simulink model "XY_2mm_accelcontrol"  (R2023a)
settings: Solver=ode1  StartTime=0.0  StopTime=inf  FixedStep=0.001  RelTol=1e-3  EnableMultiTasking=on
PostLoadFcn:
  | , if any(exist('dsrtsu_mdlpostloadfcn', 'file') ~= 0), dsrtsu_mdlpostloadfcn('Execute', bdroot); end,
InitFcn:
  | , if any(exist('rtifpga_mdlclblib', 'file') ~= 0), rtifpga_mdlclblib('Init', bdroot); end,
  | [b,a] = butter(6,0.6)
  | N_coils = 6
  | % Load mean voltage needed for stationary levitation at "center" for the ML model's given dataset
  | load("D:\Maglev_Project\00_WORKSTATION\MATLAB Training\alldata.mat","Vmean_raw")
  | tic
model workspace (MAT data in the model file):
  Iters = 5
  N_coils = 6
  fatness_default = 1
  running = 0
  z0_default = 0.080001
undefined symbols (not defined in the file or in its folder): a, b, DiscIntNeverNeededParam, Vmean_raw
libraries: neural x15, simulink x8, commfilt2 x7, dspstat3 x4, rti2004lib x3, rtilibm x1
(part 1 of 3)
settings Model: DSRTSU_INTERNAL_RTI_VER=620  DSRTSU_INTERNAL_RTI_TYPE=rti1006  DSRTSU_INTERNAL_RTIFPGA=200  DSRTSU_INTERNAL_RTISTBM_VER=23.1  Creator=Administrator  LastModifiedBy=inst
settings SolverCC: AlgebraicLoopSolver=TrustRegion
settings DataIOCC: LimitDataPoints=on  SaveFormat=Array  SignalLoggingSaveFormat=ModelDataLogs  ReturnWorkspaceOutputs=off
settings OptimizationCC: BlockReduction=off  OptimizeBlockIOStorage=off  BufferReuse=off  ReuseModelBlockBuffer=off  ExpressionFolding=off  ExpressionDepthLimit=2147483647  LocalBlockOutputs=off  LifeSpan=inf
settings DebuggingCC: UnderspecifiedInitializationDetection=Classic  MergeDetectMultiDrivingBlocksExec=none  SolverPrmCheckMsg=warning  FcnCallInpInsideContextMsg=warning  UnconnectedInputMsg=warning  UnconnectedOutputMsg=warning  UnconnectedLineMsg=warning  StateNameClashWarn=warning  SFUnexpectedBacktrackingDiag=warning  SFNoUnconditionalDefaultTransitionDiag=warning  SFExecutionAtInitializationDiag=none  ArithmeticOperatorsInVariantConditions=warning
settings HardwareCC: ProdBitPerPointer=32  ProdBitPerSizeT=32  ProdBitPerPtrDiffT=32  ProdLargestAtomicInteger=Integer  ProdWordSize=32  ProdHWDeviceType=Custom Processor->Custom  TargetIntDivRoundTo=Zero  TargetEndianess=LittleEndian  TargetHWDeviceType=Custom Processor->Custom
settings ModelReferenceCC: EnableRefExpFcnMdlSchedulingChecks=on  PropagateSignalLabelsOutOfModel=off
settings SFSimCC: SimUseLocalCustomCode=off  MATLABDynamicMemAlloc=off  CustomCodeUndefinedFunction=UseInterfaceOnly
settings RTWCC: Description=dSPACE DS1006 Hardware Platform  SystemTargetFile=rti1006.tlc  MakeCommand=make_rti  TemplateMakefile=rti1006.tmf  RTWUseLocalCustomCode=off
settings CodeAppCC: StateflowObjectComments=on
settings STFCustomTargetCC: TargetLangStandard=C89/C90 (ANSI)  ParMdlRefBuildCompliant=on  ConcurrentExecutionCompliant=off  GRTInterface=off  UseToolchainInfoCompliant=off  SystemTargetFile=rti1006.tlc
settings GRTTargetCC: TargetLangStandard=C89/C90 (ANSI)  CompOptLevelCompliant=off  ConcurrentExecutionCompliant=off  CombineOutputUpdateFcns=off  MatFileLogging=off  CPPClassGenCompliant=off  UseToolchainInfoCompliant=off  ExtModeMexFile=noextcomm
settings ConfigComp: CovMetricSettings=dw  CovSaveCumulativeToWorkspaceVar=on  CovSaveSingleToWorkspaceVar=on

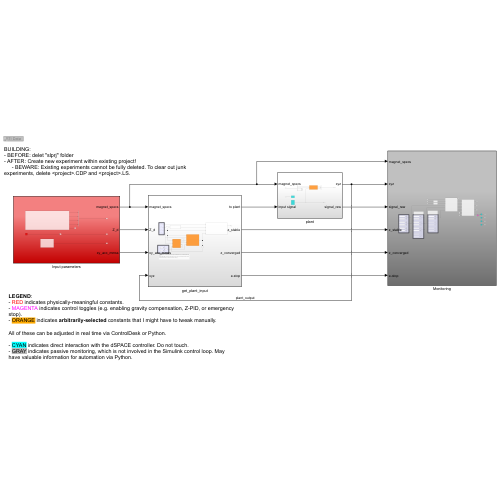
[thumbnail: Simulink's stored preview of the top-level diagram]
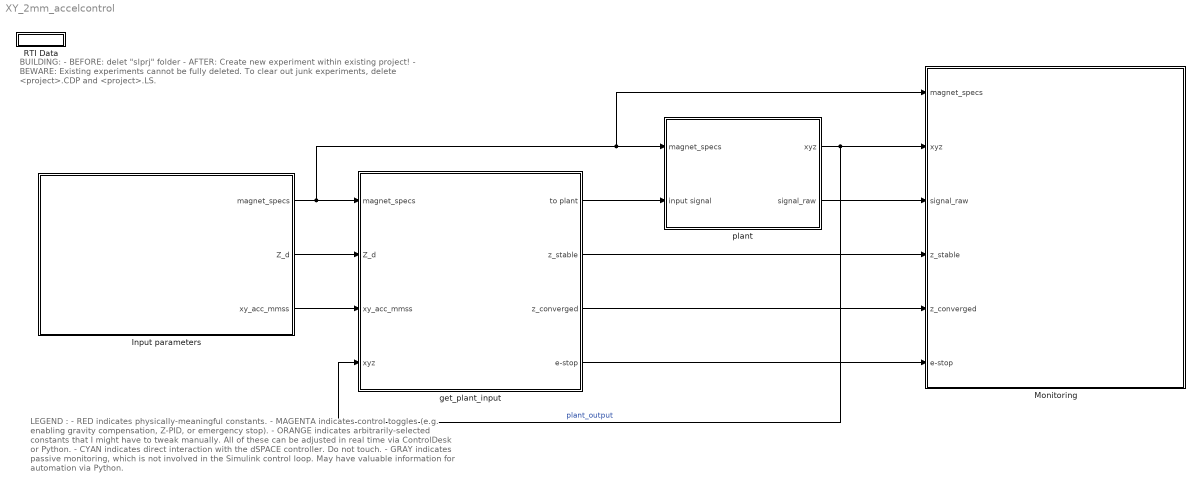
== system XY_2mm_accelcontrol ==
  note: BUILDING:
      | - BEFORE: delet "slprj" folder
      | - AFTER: Create new experiment within existing project!
      | - BEWARE: Existing experiments cannot be fully deleted. To clear out junk experiments, delete <project>.CDP and <project>.LS.
  note: LEGEND :
      | - RED indicates physically-meaningful constants.
      | - MAGENTA indicates control toggles (e.g. enabling gravity compensation, Z-PID, or emergency stop).
      | - ORANGE indicates arbitrarily-selected constants that I might have to tweak manually.
      |
      | All of these can be adjusted in real time via ControlDesk or Python.
      |
      | - CYAN indicates direct interaction with the dSPACE controller. Do not touch.
      | - GRAY indicates passive monitoring, which is not involved in the Simulink control loop. May have valuable information for automation via Python.
  Input parameters : Subsystem
  Monitoring : Subsystem
  RTI Data : Subsystem  Tag=struct('RTIDataServer',struct('RTIDataServerVs','2','RTIModelDescription','struct(''main'',''XY_2mm_accelcontrol'',''sub'','''',''isMp'',0)'))  LoadFcn="if exist('rtidc'), try,  rtidc('DataHostBlockClbLoad', gcbh); catch, disp(['Warning: ''LoadFcn'' for RTI Data block failed: ' lasterr]); end, end,"  mask(RTI_DATA_HOST){}
      mask help:
      | RTI Data Block.
      | This block is used by RTI to store internal model-dependent data.
      | Please keep this block on the root level of the model. Deleting this block will result in data loss.
      |
      | NEVER DELETE OR COPY THIS BLOCK!
      settings: CopyFcn="if exist('rtidc'), try,  rtidc('DataHostBlockClbCopy', gcbh); catch, disp(['Warning: ''CopyFcn'' for RTI Data block failed: ' lasterr]); end, end,"  DeleteFcn="if exist('rtidc'), try,  rtidc('DataHostBlockClbDelete', gcbh); catch, disp(['Warning: ''DeleteFcn'' for RTI Data block failed: ' lasterr]); end, end,"  ModelCloseFcn="if exist('rtidc'), try,  rtidc('DataHostBlockClbModelClose', gcbh); catch, disp(['Warning: ''ModelCloseFcn'' for RTI Data block failed: ' lasterr]); end, end,"  PreSaveFcn="if exist('rtidc'), try,  rtidc('DataHostBlockClbPreSave', gcbh); catch, disp(['Warning: ''PreSaveFcn'' for RTI Data block failed: ' lasterr]); end, end,"  PostSaveFcn="if exist('rtidc'), try,  rtidc('DataHostBlockClbPostSave', gcbh); catch, disp(['Warning: ''PostSaveFcn'' for RTI Data block failed: ' lasterr]); end, end,"  NameChangeFcn="if exist('rtidc'), try,  rtidc('DataHostBlockClbNameChange', gcbh); catch, disp(['Warning: ''NameChangeFcn'' for RTI Data block failed: ' lasterr]); end, end,"
      mask Help:
      | RTI Data Block.
      | This block is used by RTI to store internal model-dependent data.
      | Please keep this block on the root level of the model. Deleting this block will result in data loss.
      | 
      | NEVER DELETE OR COPY THIS BLOCK!
      mask Display:
      | text(0.5, 0.5, 'RTI Data', 'HorizontalAlignment', 'center');
      | plot([1 0]);
  get_plant_input : Subsystem
  plant : Subsystem
  wires:
  Input parameters/1(magnet_specs) -> Monitoring/1(magnet_specs), plant/1(magnet_specs), get_plant_input/1(magnet_specs)
  Input parameters/2(Z_d) -> get_plant_input/2(Z_d)
  plant/1(xyz) -> get_plant_input/4(xyz), Monitoring/2(xyz)  "plant_output"
  Input parameters/3(xy_acc_mmss) -> get_plant_input/3(xy_acc_mmss)
  get_plant_input/1(to plant) -> plant/2(input signal)
  plant/2(signal_raw) -> Monitoring/3(signal_raw)
  get_plant_input/2(z_stable) -> Monitoring/4(z_stable)
  get_plant_input/3(z_converged) -> Monitoring/5(z_converged)
  get_plant_input/4(e-stop) -> Monitoring/6(e-stop)

== system XY_2mm_accelcontrol/Input parameters ==
  Acceleration input : Subsystem
  Magnet Specs : Subsystem
  Mux : Mux
  Terminator : Terminator
  Z_desired_true : Constant  Value=0
  gain_dummy : Gain
  magnet_specs : Outport
  Z_d : Outport  Port=2
  xy_acc_mmss : Outport  Port=3
  wires:
  Magnet Specs/1(diameter_m) -> Mux/1
  Magnet Specs/2(height_m) -> Mux/2
  Magnet Specs/3(mass_g) -> Mux/3
  Magnet Specs/4(B_r) -> Mux/4
  Mux/1 -> magnet_specs/1
  Magnet Specs/5(errorflag) -> Terminator/1
  Z_desired_true/1 -> gain_dummy/1  "Z_d_true_test_inputparameters"
  gain_dummy/1 -> Z_d/1  "Z_d_test_dummygain"
  Acceleration input/1(xy_acc_mmss) -> xy_acc_mmss/1

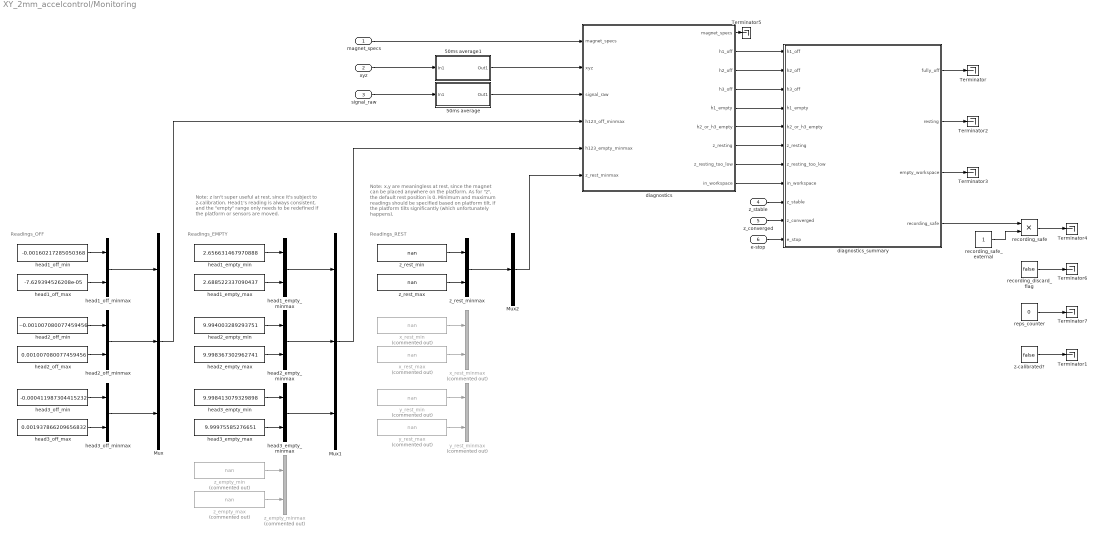
== system XY_2mm_accelcontrol/Monitoring ==
  note: Note: x,y are meaningless at rest, since the magnet can be placed anywhere on the platform.
      |
      | As for "z", the default rest position is 0. Minimum and maximum readings should be specified based on platform tilt, if the platform tilts significantly (which unfortunately happens).
  note: Readings_OFF
  note: Readings_REST
  note: Readings_EMPTY
  note: Note: z isn't super useful at rest, since it's subject to z-calibration.
      | Head1's reading is always consistent, and the "empty" range only needs to be redefined if the platform or sensors are moved.
  magnet_specs : Inport
  xyz : Inport  Port=2
  signal_raw : Inport  Port=3
  z_stable : Inport  Port=4
  z_converged : Inport  Port=5
  e-stop : Inport  Port=6
  50ms average : Subsystem
  50ms average1 : Subsystem
  Mux : Mux  Inputs=3
  Mux1 : Mux  Inputs=3
  Mux2 : Mux  Inputs=1
  Terminator{,1..7} (8 alike) : Terminator
  diagnostics : MATLAB Function  TreatAsAtomicUnit=on
  diagnostics_summary : MATLAB Function  TreatAsAtomicUnit=on
  head1_empty_max : Constant  Value=2.688522337090437
  head1_empty_min : Constant  Value=2.656631467970888
  head1_empty_minmax : Mux  Inputs=2
  head1_off_max : Constant  Value=-7.629394526208e-05
  head1_off_min : Constant  Value=-0.00160217285050368
  head1_off_minmax : Mux  Inputs=2
  head2_empty_max : Constant  Value=9.998367302962741
  head2_empty_min : Constant  Value=9.994003289293751
  head2_empty_minmax : Mux  Inputs=2
  head2_off_max : Constant  Value=0.001007080077459456
  head2_off_min : Constant  Value=--0.001007080077459456
  head2_off_minmax : Mux  Inputs=2
  head3_empty_max : Constant  Value=9.99975585276651
  head3_empty_min : Constant  Value=9.998413079329898
  head3_empty_minmax : Mux  Inputs=2
  head3_off_max : Constant  Value=0.001937866209656832
  head3_off_min : Constant  Value=-0.000411987304415232
  head3_off_minmax : Mux  Inputs=2
  recording_discard_flag : Constant  Value=false
  recording_safe : Product
  recording_safe_external : Constant
  reps_counter : Constant  Value=0
  x_rest_max : Constant  Commented=on  Value=nan
  x_rest_min : Constant  Commented=on  Value=nan
  x_rest_minmax : Mux  Commented=on  Inputs=2
  y_rest_max : Constant  Commented=on  Value=nan
  y_rest_min : Constant  Commented=on  Value=nan
  y_rest_minmax : Mux  Commented=on  Inputs=2
  z-calibrated? : Constant  Value=false
  z_empty_max : Constant  Commented=on  Value=nan
  z_empty_min : Constant  Commented=on  Value=nan
  z_empty_minmax : Mux  Commented=on  Inputs=2
  z_rest_max : Constant  Value=nan
  z_rest_min : Constant  Value=nan
  z_rest_minmax : Mux  Inputs=2
  wires:
  head1_off_min/1 -> head1_off_minmax/1
  head1_off_max/1 -> head1_off_minmax/2
  head2_off_min/1 -> head2_off_minmax/1
  head2_off_max/1 -> head2_off_minmax/2
  head3_off_max/1 -> head3_off_minmax/2
  head3_off_min/1 -> head3_off_minmax/1
  x_rest_max/1 -> x_rest_minmax/2
  z_rest_min/1 -> z_rest_minmax/1
  z_rest_max/1 -> z_rest_minmax/2
  y_rest_max/1 -> y_rest_minmax/2
  x_rest_min/1 -> x_rest_minmax/1
  y_rest_min/1 -> y_rest_minmax/1
  head3_empty_min/1 -> head3_empty_minmax/1
  head2_empty_min/1 -> head2_empty_minmax/1
  head3_empty_max/1 -> head3_empty_minmax/2
  head1_empty_min/1 -> head1_empty_minmax/1
  head2_empty_max/1 -> head2_empty_minmax/2
  head1_empty_max/1 -> head1_empty_minmax/2
  head1_off_minmax/1 -> Mux/1
  head2_off_minmax/1 -> Mux/2
  head3_off_minmax/1 -> Mux/3
  head2_empty_minmax/1 -> Mux1/2
  head3_empty_minmax/1 -> Mux1/3
  head1_empty_minmax/1 -> Mux1/1
  z_rest_minmax/1 -> Mux2/1
  Mux/1 -> diagnostics/4(h123_off_minmax)
  Mux1/1 -> diagnostics/5(h123_empty_minmax)
  Mux2/1 -> diagnostics/6(z_rest_minmax)
  z_empty_max/1 -> z_empty_minmax/2
  z_empty_min/1 -> z_empty_minmax/1
  magnet_specs/1 -> diagnostics/1("magnet_specs ")
  xyz/1 -> 50ms average1/1(In1)
  signal_raw/1 -> 50ms average/1(In1)
  z-calibrated?/1 -> Terminator1/1
  50ms average/1(Out1) -> diagnostics/3(signal_raw)
  50ms average1/1(Out1) -> diagnostics/2(xyz)
  diagnostics/2(h1_off) -> diagnostics_summary/1(h1_off)
  diagnostics/3(h2_off) -> diagnostics_summary/2(h2_off)
  diagnostics/4(h3_off) -> diagnostics_summary/3(h3_off)
  diagnostics/5(h1_empty) -> diagnostics_summary/4(h1_empty)
  diagnostics/6(h2_or_h3_empty) -> diagnostics_summary/5(h2_or_h3_empty)
  diagnostics/1(magnet_specs) -> Terminator5/1
  diagnostics/7(z_resting) -> diagnostics_summary/6(z_resting)
  diagnostics/8(z_resting_too_low) -> diagnostics_summary/7(z_resting_too_low)
  diagnostics/9(in_workspace) -> diagnostics_summary/8(in_workspace)
  diagnostics_summary/1(fully_off) -> Terminator/1
  diagnostics_summary/2(resting) -> Terminator2/1
  diagnostics_summary/3(empty_workspace) -> Terminator3/1
  diagnostics_summary/4(recording_safe) -> recording_safe/1
  z_converged/1 -> diagnostics_summary/10(z_converged)
  e-stop/1 -> diagnostics_summary/11(e_stop)
  recording_safe_external/1 -> recording_safe/2
  recording_safe/1 -> Terminator4/1
  z_stable/1 -> diagnostics_summary/9(z_stable)
  recording_discard_flag/1 -> Terminator6/1
  reps_counter/1 -> Terminator7/1

== system XY_2mm_accelcontrol/RTI Data ==
  RTI Data Store : Subsystem  Tag="struct('private',struct('version',struct('dsVer',uint32(2),'dsVerCreation',uint32(2),'RTI',struct('ver','6.2','type','RTI1006')),'access',struct('type','Model','isPerm',1,'created',['29-Jul-2010 10:53:51'],'modified',['20-Nov-2024 19:17:44'],'location','')),'public',struct('main',struct('data',[]),'sub',struct('name',{{'XY_2mm_accelcontrol'}},'data',{{struct('TH',struct('thTaskInfo',struct('taskType',{'TIMER','HWINT','TMRINT','SWINT','GLINT'},'tasksNumOf',{1,0,0,0,0},'srcIds',{{'TIMERA'},{},{},{},{}},'taskNames',{{['Timer Task 1']},{},{},{},{}})),'th_tc',struct('dataType','TASK','taskGroupId','','taskGroupList',{{}},'taskSchedulingPolicy','FCFS','taskType','TIMER','blkh',-1,'srcId','TIMERA','srcSgnName',['Timer A interrupt'],'srcCpuName','','taskName',['Timer Task 1  [0.001] s'],'taskNameDisplayExt','','smplTime',0.001,'smplTimeOffs',0,'hasFixedPriority',0,'priority',1,'hasFixedOvc',0,'ovcType',1,'ovcMax',1),'tc_th',struct('dataType','TASK','taskGroupId','','taskGroupList',{{}},'taskSchedulingPolicy','FCFS','taskType','TIMER','blkh',-1,'srcId','TIMERA','srcSgnName',['Timer A interrupt'],'srcCpuName','','taskName',['Timer Task 1  [0.001] s'],'taskNameDisplayExt','','smplTime',0.001,'smplTimeOffs',0,'hasFixedPriority',0,'priority',1,'hasFixedOvc',0,'ovcType',1,'ovcMax',1))}})))"  mask(RTI_DATA_STORE){}
      mask help:
      | RTI Data Store Block. This block is used by RTI to store internal model dependent data. Deleting this block will result in data loss.
      |
      | NEVER DELETE, COPY, OR MODIFY THIS BLOCK!
      mask Help:
      | RTI Data Store Block. This block is used by RTI to store internal model dependent data. Deleting this block will result in data loss.
      | 
      | NEVER DELETE, COPY, OR MODIFY THIS BLOCK!
      mask Display: text(0.5, 0.5, ' ', 'HorizontalAlignment', 'center');

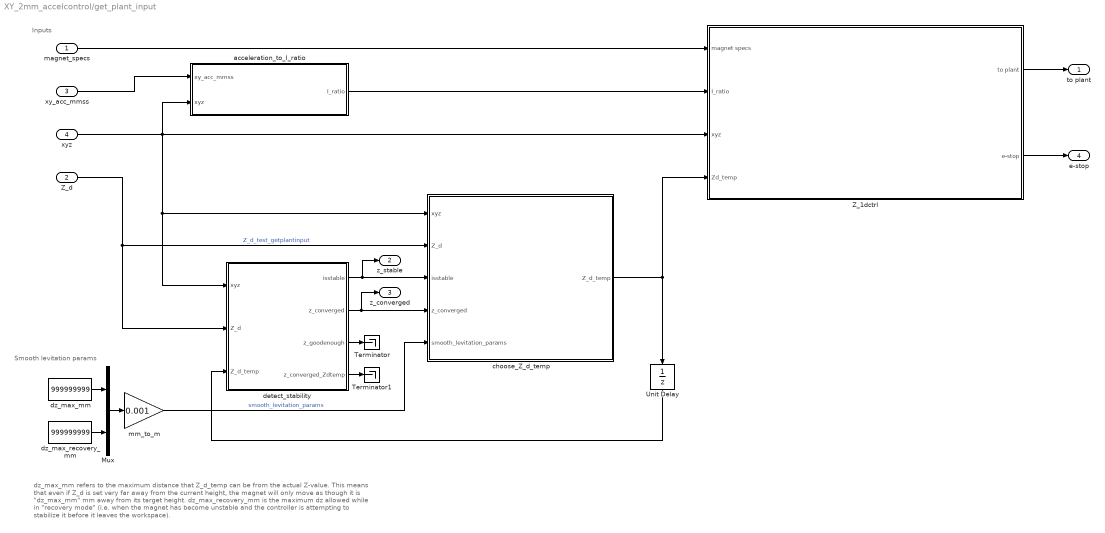
== system XY_2mm_accelcontrol/get_plant_input ==
  note: dz_max_mm refers to the maximum distance that Z_d_temp can be from the actual Z-value. This means that even if Z_d is set very far away from the current height, the magnet will only move as though it is "dz_max_mm" mm away from its target height.
      |
      | dz_max_recovery_mm is the maximum dz allowed while in "recovery mode" (i.e. when the magnet has become unstable and the controller is attempting to stabilize it before it leaves the workspace).
  note: Smooth levitation params
  note: Inputs
  magnet_specs : Inport
  Z_d : Inport  Port=2
  xy_acc_mmss : Inport  Port=3
  xyz : Inport  Port=4
  Mux : Mux  Inputs=2
  Terminator : Terminator
  Terminator1 : Terminator
  Unit Delay : UnitDelay  SampleTime=-1  HasFrameUpgradeWarning=on
  Z_1dctrl : Subsystem
  acceleration_to_I_ratio : Subsystem
  choose_Z_d_temp : Subsystem
  detect_stability : Subsystem
  dz_max_mm : Constant  Value=999999999
  dz_max_recovery_mm : Constant  Value=999999999
  mm_to_m : Gain  Gain=0.001
  to plant : Outport
  z_stable : Outport  Port=2
  z_converged : Outport  Port=3
  e-stop : Outport  Port=4
  wires:
  Z_d/1 -> detect_stability/2(Z_d), choose_Z_d_temp/2(Z_d)  "Z_d_test_getplantinput"
  xyz/1 -> acceleration_to_I_ratio/2(xyz), Z_1dctrl/3(xyz), detect_stability/1(xyz), choose_Z_d_temp/1(xyz)
  detect_stability/1(isstable) -> z_stable/1, choose_Z_d_temp/3(isstable)
  dz_max_mm/1 -> Mux/1
  dz_max_recovery_mm/1 -> Mux/2
  Mux/1 -> mm_to_m/1
  choose_Z_d_temp/1(Z_d_temp) -> Z_1dctrl/4(Zd_temp), Unit Delay/1
  detect_stability/2(z_converged) -> z_converged/1, choose_Z_d_temp/4(z_converged)
  detect_stability/3(z_goodenough) -> Terminator/1
  Unit Delay/1 -> detect_stability/3(Z_d_temp)
  Z_1dctrl/1(to plant) -> to plant/1
  magnet_specs/1 -> Z_1dctrl/1(magnet specs)
  xy_acc_mmss/1 -> acceleration_to_I_ratio/1(xy_acc_mmss)
  mm_to_m/1 -> choose_Z_d_temp/5(smooth_levitation_params)  "smooth_levitation_params"
  detect_stability/4(z_converged_Zdtemp) -> Terminator1/1
  Z_1dctrl/2(e-stop) -> e-stop/1
  acceleration_to_I_ratio/1(I_ratio) -> Z_1dctrl/2(I_ratio)

== system XY_2mm_accelcontrol/plant ==
  magnet_specs : Inport  PortDimensions=[1 4]
  input signal : Inport  Port=2
  DS2103_B1 : rtilibm/DS2103/DS2103_B1  BoardNo=1  ChannelNos=[1 2 4 6 8 9 10 11 12 18 19 20]  Range=[10 10 10 10 10 10 10 10 10 10 10 10 10 10 10 10 10 10 10 10 10 10 10 10 10 10 10 10 10 10 10 10]  IOErrorMode=[1 1 1 1 1 1 1 1]  InitValue=[0 0 0 0 0 0 0 0 0 0 0 0 0 0 0 0 0 0 0 0 0 0 0 0 0 0 0 0 0 0 0 0]  TermMode=[0 0 0 0 0 0 0 1 1 1 1 1 1 1 1 1 1 1 1 1 1 1 1 1 1 1 1 1 1 1 1 1]  TermValue=[0 0 0 0 0 0 0 0 0 0 0 0 0 0 0 0 0 0 0 0 0 0 0 0 0 0 0 0 0 0 0 0]  DialogFcn=gui2103  UnitName={ 'DS2103_B' }  UnitValues={ 1 }  DSProperties=struct('RTI',struct('Version',uint32(1),'BlockType',struct('isSLSource',uint8(0),'isSLSink',uint8(1),'isHWSource',uint8(0),'isHWSink',uint8(1),'isSetup',uint8(0),'isInline',uint8(1),'isNonInline',uint8(0),'isInterrupt',uint8(0),'isChannelwise',uint8(0)),'IOBoardType','DS2103','UnitType','DAC','Identifier','DACMUX','DialogType','ML','BlockSet','NONE','SlaveProcessor','NONE'))
      settings: SourceProductName=dSPACE RTI1006
  Demux : Demux
  Mux : Mux  Inputs=3
  Position Determination1 : Subsystem  TreatAsAtomicUnit=on
  Terminator : Terminator
  Terminator2 : Terminator
  output signal : Subsystem
  xyz : Outport
  signal_raw : Outport  Port=2
  wires:
  input signal/1 -> DS2103_B1/1
  Demux/4 -> Terminator/1  "B_r"
  Demux/1 -> Position Determination1/1(height_m)  "diameter_m"
  Demux/2 -> Position Determination1/2(diameter_m)  "height_m"
  Demux/3 -> Terminator2/1  "mass_g"
  Position Determination1/1(X(m)) -> Mux/1  "x_pos"
  Position Determination1/2(Y(m)) -> Mux/2  "y_pos"
  Position Determination1/3(Z(m)) -> Mux/3  "z_pos"
  output signal/1(plant signals) -> signal_raw/1, Position Determination1/3(plant signals)
  Mux/1 -> xyz/1
  magnet_specs/1 -> Demux/1

== system XY_2mm_accelcontrol/Input parameters/Acceleration input ==
  MATLAB Function : MATLAB Function  TreatAsAtomicUnit=on
  Mux : Mux  Inputs=2
  Terminator : Terminator
  Units_mode : Constant
  x_acc : Constant  Value=0
  y_acc : Constant  Value=0
  xy_acc_mmss : Outport
  wires:
  Units_mode/1 -> MATLAB Function/1(unit_mode)  "unit_mode"
  y_acc/1 -> MATLAB Function/3(y_acc)
  x_acc/1 -> MATLAB Function/2(x_acc)
  MATLAB Function/1(x_acc_mmss) -> Mux/1
  MATLAB Function/2(y_acc_mmss) -> Mux/2
  Mux/1 -> xy_acc_mmss/1
  MATLAB Function/3(errorflag) -> Terminator/1

== system XY_2mm_accelcontrol/Input parameters/Magnet Specs ==
  note: NOTE: Xiaodong lists the magnet as having 10mm height and 10mm diameter. However, height is closer to 11-12mm. Diameter is closer to ????.
  Diameter : Constant  Value=0.635
  Height : Constant  Value=0.635
  Magnet Physical Specs : MATLAB Function  TreatAsAtomicUnit=on
  Mass (g) : Constant  Value=1.5081
  Units : StringConstant  Commented=on  String="\"cm\""
  Units_mode : Constant  Value=2
  mag-field Br value (in T or G) : Constant  Value=1.45
  string to unit mode : Subsystem  Commented=on
  diameter_m : Outport
  height_m : Outport  Port=2
  mass_g : Outport  Port=3
  B_r : Outport  Port=4
  errorflag : Outport  Port=5
  wires:
  Diameter/1 -> Magnet Physical Specs/2(diameter)
  Height/1 -> Magnet Physical Specs/3(height)
  Mass (g)/1 -> Magnet Physical Specs/4(mass)
  Magnet Physical Specs/1(diameter_m) -> diameter_m/1
  Magnet Physical Specs/2(height_m) -> height_m/1
  Magnet Physical Specs/4(B_r) -> B_r/1
  Magnet Physical Specs/3(mass_g) -> mass_g/1
  Magnet Physical Specs/5(errorflag) -> errorflag/1
  Units_mode/1 -> Magnet Physical Specs/1(unit_mode)  "unit_mode"
  mag-field Br value (in T or G)/1 -> Magnet Physical Specs/5(magnet_remanence_t)
  Units/1 -> string to unit mode/1(In1)

== system XY_2mm_accelcontrol/Monitoring/50ms average ==
  In1 : Inport
  ave z : Product  Inputs=*/
  integration window (samples) : Constant  Value=50
  sum of z over short time : commfilt2/Windowed Integrator  integperiod=50  roundingMode=Floor  overflowMode=off  coeffDataTypeStr=Inherit: Same word length as input  coeffMin=[]  coeffMax=[]  coeffLastDataTypeStr=Inherit: Same word length as input  accumDataTypeStr=Inherit: Same as product output  accumLastDataTypeStr=Inherit: Same as product output  outputDataTypeStr=Inherit: Same as accumulator  outputMin=[]  outputMax=[]  outputLastDataTypeStr=Inherit: Same as accumulator
  Out1 : Outport
  wires:
  integration window (samples)/1 -> ave z/2
  In1/1 -> sum of z over short time/1
  sum of z over short time/1 -> ave z/1
  ave z/1 -> Out1/1

== system XY_2mm_accelcontrol/Monitoring/50ms average1 ==
  In1 : Inport
  ave z : Product  Inputs=*/
  integration window (samples) : Constant  Value=50
  sum of z over short time : commfilt2/Windowed Integrator  integperiod=50  roundingMode=Floor  overflowMode=off  coeffDataTypeStr=Inherit: Same word length as input  coeffMin=[]  coeffMax=[]  coeffLastDataTypeStr=Inherit: Same word length as input  accumDataTypeStr=Inherit: Same as product output  accumLastDataTypeStr=Inherit: Same as product output  outputDataTypeStr=Inherit: Same as accumulator  outputMin=[]  outputMax=[]  outputLastDataTypeStr=Inherit: Same as accumulator
  Out1 : Outport
  wires:
  integration window (samples)/1 -> ave z/2
  In1/1 -> sum of z over short time/1
  sum of z over short time/1 -> ave z/1
  ave z/1 -> Out1/1

== system XY_2mm_accelcontrol/RTI Data/RTI Data Store ==
  RTI Data Store : Subsystem  mask(RTI_DATA_STORE){}
      mask help:
      | RTI Data Store Block. This block is used by RTI to store internal model dependent data. Deleting this block will result in data loss.
      |
      | NEVER DELETE, COPY, OR MODIFY THIS BLOCK!
      mask Help:
      | RTI Data Store Block. This block is used by RTI to store internal model dependent data. Deleting this block will result in data loss.
      | 
      | NEVER DELETE, COPY, OR MODIFY THIS BLOCK!
      mask Display: text(0.5, 0.5, ' ', 'HorizontalAlignment', 'center');

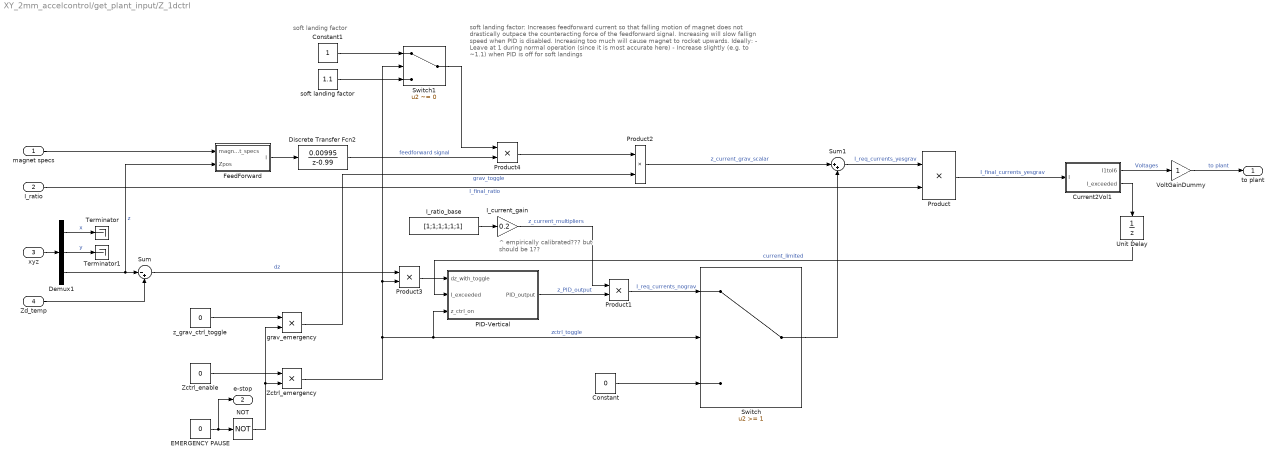
== system XY_2mm_accelcontrol/get_plant_input/Z_1dctrl ==
  note: soft landing factor
  note: ^ empirically calibrated???
      | but should be 1??
  note: soft landing factor:
      | Increases feedforward current so that falling motion of magnet does not drastically outpace the counteracting force of the feedforward signal.
      | Increasing will slow fallign speed when PID is disabled. Increasing too much will cause magnet to rocket upwards.
      |
      | Ideally:
      | - Leave at 1 during normal operation (since it is most accurate here)
      | - Increase slightly (e.g. to ~1.1) when PID is off for soft landings
  magnet specs : Inport
  I_ratio : Inport  Port=2
  xyz : Inport  Port=3
  Zd_temp : Inport  Port=4
  Constant : Constant  Value=0
  Constant1 : Constant
  Current2Vol1 : Subsystem  TreatAsAtomicUnit=on
  Demux1 : Demux  Outputs=3
  Discrete Transfer Fcn2 : DiscreteTransferFcn  Numerator=[0.00995]  Denominator=[1 -0.99]
  EMERGENCY PAUSE : Constant  Value=0
  FeedForward : Subsystem  TreatAsAtomicUnit=on
  I_current_gain : Gain  Gain=0.2
  I_ratio_base : Constant  Value=[1;1;1;1;1;1]
  NOT : Logic  Operator=NOT  IconShape=distinctive  AllPortsSameDT=off  OutDataTypeStr=boolean
  PID-Vertical : Subsystem  TreatAsAtomicUnit=on
  Product{,1..4} (5 alike) : Product
  Sum : Sum  Inputs=|-+
  Sum1 : Sum  Inputs=|++
  Switch : Switch  Threshold=1  SaturateOnIntegerOverflow=off  InputSameDT=off
  Switch1 : Switch  Criteria=u2 ~= 0  Threshold=1  SaturateOnIntegerOverflow=off  InputSameDT=off
  Terminator : Terminator
  Terminator1 : Terminator
  Unit Delay : UnitDelay  InitialCondition=1  SampleTime=-1  HasFrameUpgradeWarning=on
  VoltGainDummy : Gain
  Zctrl_emergency : Product
  Zctrl_enable : Constant  Value=0
  grav_emergency : Product
  soft landing factor : Constant  Value=1.1
  z_grav_ctrl_toggle : Constant  Value=0
  to plant : Outport
  e-stop : Outport  Port=2
  wires:
  Sum/1 -> Product3/1  "dz"
  Product/1 -> Current2Vol1/1(I)  "I_final_currents_yesgrav"
  Switch/1 -> Sum1/2
  Unit Delay/1 -> PID-Vertical/2(I_exceeded)  "current_limited"
  I_ratio_base/1 -> I_current_gain/1
  z_grav_ctrl_toggle/1 -> grav_emergency/1
  Zctrl_enable/1 -> Zctrl_emergency/1
  NOT/1 -> Zctrl_emergency/2, grav_emergency/2
  Zctrl_emergency/1 -> Switch/2, PID-Vertical/3(z_ctrl_on), Switch1/2, Product3/2  "zctrl_toggle"
  grav_emergency/1 -> Product2/2  "grav_toggle"
  VoltGainDummy/1 -> to plant/1  "to plant"
  Current2Vol1/1(I1toI6) -> VoltGainDummy/1  "Voltages"
  Current2Vol1/2(I_exceeded) -> Unit Delay/1
  Product2/1 -> Sum1/1  "z_current_grav_scalar"
  I_current_gain/1 -> Product1/1  "z_current_multipliers"
  EMERGENCY PAUSE/1 -> e-stop/1, NOT/1
  Constant/1 -> Switch/3
  FeedForward/1(I) -> Discrete Transfer Fcn2/1
  Product1/1 -> Switch/1  "I_req_currents_nograv"
  Sum1/1 -> Product/1  "I_req_currents_yesgrav"
  I_ratio/1 -> Product/2  "I_final_ratio"
  PID-Vertical/1(PID_output) -> Product1/2  "z_PID_output"
  Discrete Transfer Fcn2/1 -> Product4/2  "feedforward signal"
  xyz/1 -> Demux1/1
  Demux1/2 -> Terminator1/1  "y"
  Demux1/1 -> Terminator/1  "x"
  magnet specs/1 -> FeedForward/1(magnet_specs)
  Demux1/3 -> FeedForward/2(Zpos), Sum/1  "z"
  Zd_temp/1 -> Sum/2
  Product3/1 -> PID-Vertical/1(dz_with_toggle)
  Product4/1 -> Product2/1
  Constant1/1 -> Switch1/1
  soft landing factor/1 -> Switch1/3
  Switch1/1 -> Product4/1

== system XY_2mm_accelcontrol/get_plant_input/acceleration_to_I_ratio ==
  note: ^--
      | Does this need a filter for smoothing?
  xy_acc_mmss : Inport
  xyz : Inport  Port=2
  Actually apply voltages : Subsystem
  Demux1 : Demux  Outputs=3
  Make ratios add up to 1 : Subsystem  TreatAsAtomicUnit=on
  Mux : Mux  Inputs=2
  Number of coils : Gain  Gain=N_coils
  Terminator2 : Terminator
  Voltages from ML : Subsystem
  m_to_mm : Gain  Gain=1000
  I_ratio : Outport
  wires:
  Voltages from ML/1(Voltages) -> Actually apply voltages/1(Voltages)
  Number of coils/1 -> I_ratio/1  "I_final_ratio"
  Make ratios add up to 1/1(Voltage_ratio) -> Number of coils/1  "I_ratio_norm"
  Demux1/1 -> Mux/1  "x"
  xyz/1 -> Demux1/1
  Demux1/2 -> Mux/2  "y"
  Demux1/3 -> Terminator2/1  "z"
  Mux/1 -> m_to_mm/1
  m_to_mm/1 -> Voltages from ML/2(xy_mm)
  xy_acc_mmss/1 -> Voltages from ML/1(xy_acc_mmss)
  Actually apply voltages/1(Out1) -> Make ratios add up to 1/1(Voltages)

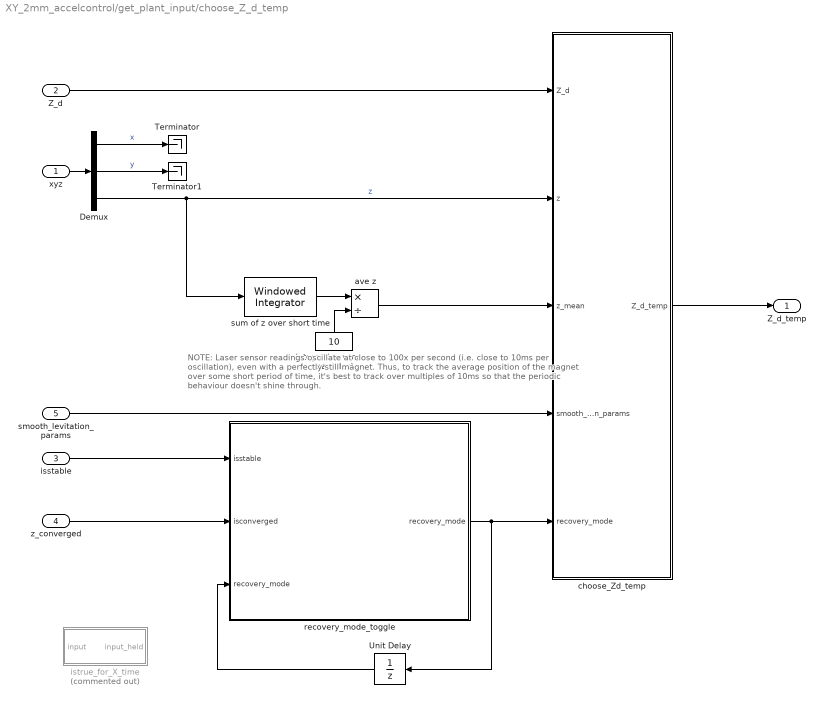
== system XY_2mm_accelcontrol/get_plant_input/choose_Z_d_temp ==
  note: NOTE:
      | Laser sensor readings oscillate at close to 100x per second (i.e. close to 10ms per oscillation), even with a perfectly still magnet.
      | Thus, to track the average position of the magnet over some short period of time, it's best to track over multiples of 10ms so that the periodic behaviour doesn't shine through.
  xyz : Inport
  Z_d : Inport  Port=2
  isstable : Inport  Port=3
  z_converged : Inport  Port=4
  smooth_levitation_params : Inport  Port=5
  Demux : Demux  Outputs=3
  Terminator : Terminator
  Terminator1 : Terminator
  Unit Delay : UnitDelay  InitialCondition=5  SampleTime=-1  HasFrameUpgradeWarning=on
  ave z : Product  Inputs=*/
  choose_Zd_temp : MATLAB Function  TreatAsAtomicUnit=on
  integration window (samples) : Constant  Value=10
  istrue_for_X_time : Subsystem  Commented=on
  recovery_mode_toggle : MATLAB Function  TreatAsAtomicUnit=on
  sum of z over short time : commfilt2/Windowed Integrator  integperiod=10  InputProcessing=Columns as channels (frame based)  roundingMode=Floor  overflowMode=off  coeffDataTypeStr=Inherit: Same word length as input  coeffMin=[]  coeffMax=[]  coeffLastDataTypeStr=Inherit: Same word length as input  accumDataTypeStr=Inherit: Same as product output  accumLastDataTypeStr=Inherit: Same as product output  outputDataTypeStr=Inherit: Same as accumulator  outputMin=[]  outputMax=[]  outputLastDataTypeStr=Inherit: Same as accumulator
  Z_d_temp : Outport
  wires:
  isstable/1 -> recovery_mode_toggle/1(isstable)
  z_converged/1 -> recovery_mode_toggle/2(isconverged)
  Demux/2 -> Terminator1/1  "y"
  xyz/1 -> Demux/1
  Demux/1 -> Terminator/1  "x"
  Unit Delay/1 -> recovery_mode_toggle/3("recovery_mode ")
  Z_d/1 -> choose_Zd_temp/1(Z_d)
  Demux/3 -> sum of z over short time/1, choose_Zd_temp/2(z)  "z"
  choose_Zd_temp/1(Z_d_temp) -> Z_d_temp/1
  smooth_levitation_params/1 -> choose_Zd_temp/4(smooth_levitation_params)
  recovery_mode_toggle/1(recovery_mode) -> Unit Delay/1, choose_Zd_temp/5(recovery_mode)
  integration window (samples)/1 -> ave z/2
  ave z/1 -> choose_Zd_temp/3(z_mean)
  sum of z over short time/1 -> ave z/1

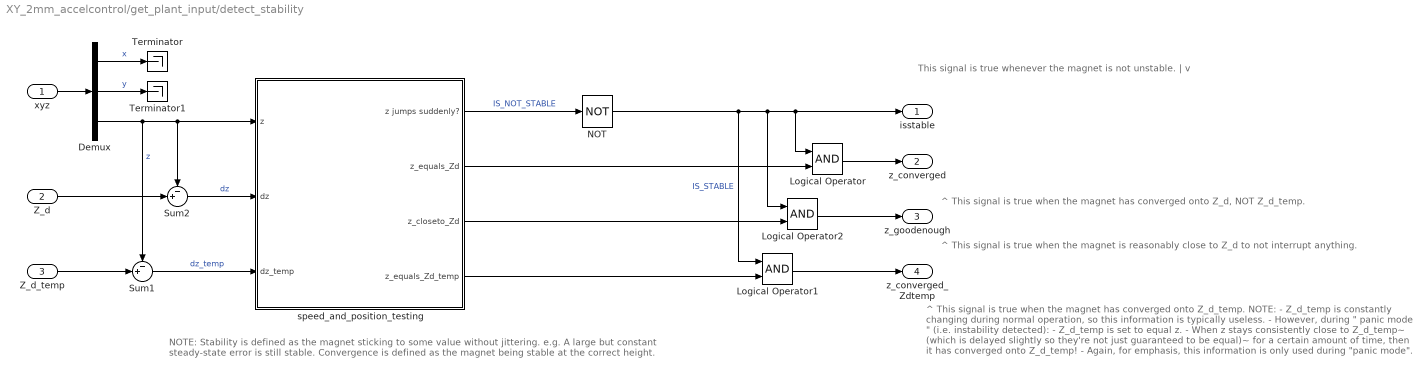
== system XY_2mm_accelcontrol/get_plant_input/detect_stability ==
  note: NOTE:
      | Stability is defined as the magnet sticking to some value without jittering. e.g. A large but constant steady-state error is still stable.
      | Convergence is defined as the magnet being stable at the correct height.
  note: This signal is true whenever the magnet is not unstable.
      | |
      | v
  note: ^ This signal is true when the magnet has converged onto Z_d, NOT Z_d_temp.
  note: ^ This signal is true when the magnet has converged onto Z_d_temp.
      |
      | NOTE:
      | - Z_d_temp is constantly changing during normal operation, so this information is typically useless.
      | - However, during " panic mode " (i.e. instability detected):
      | - Z_d_temp is set to equal z.
      | - When z stays consistently close to Z_d_temp~ (which is delayed slightly so they're not just
      | guaranteed to be equal)~ for a certain amount of time, then it has converged onto Z_d_temp!
      | - Again, for emphasis, this information is only used during "panic mode".
  note: ^ This signal is true when the magnet is reasonably close to Z_d to not interrupt anything.
  xyz : Inport
  Z_d : Inport  Port=2
  Z_d_temp : Inport  Port=3
  Demux : Demux  Outputs=3
  Logical Operator : Logic  AllPortsSameDT=off  OutDataTypeStr=boolean
  Logical Operator1 : Logic  AllPortsSameDT=off  OutDataTypeStr=boolean
  Logical Operator2 : Logic  AllPortsSameDT=off  OutDataTypeStr=boolean
  NOT : Logic  Operator=NOT  IconShape=distinctive  AllPortsSameDT=off  OutDataTypeStr=boolean
  Sum1 : Sum  Inputs=-+|
  Sum2 : Sum  Inputs=-+|
  Terminator : Terminator
  Terminator1 : Terminator
  speed_and_position_testing : Subsystem  TreatAsAtomicUnit=on
  isstable : Outport
  z_converged : Outport  Port=2
  z_goodenough : Outport  Port=3
  z_converged_Zdtemp : Outport  Port=4
  wires:
  speed_and_position_testing/1(z jumps suddenly?) -> NOT/1  "IS_NOT_STABLE"
  xyz/1 -> Demux/1
  Demux/1 -> Terminator/1  "x"
  Demux/2 -> Terminator1/1  "y"
  Demux/3 -> Sum2/1, speed_and_position_testing/1(z), Sum1/1  "z"
  Z_d/1 -> Sum2/2
  NOT/1 -> Logical Operator1/1, Logical Operator2/1, isstable/1, Logical Operator/1  "IS_STABLE"
  speed_and_position_testing/2(z_equals_Zd) -> Logical Operator/2
  Logical Operator/1 -> z_converged/1
  Z_d_temp/1 -> Sum1/2
  Logical Operator1/1 -> z_converged_Zdtemp/1
  Sum2/1 -> speed_and_position_testing/2(dz)  "dz"
  Sum1/1 -> speed_and_position_testing/3(dz_temp)  "dz_temp"
  speed_and_position_testing/3(z_closeto_Zd) -> Logical Operator2/2
  speed_and_position_testing/4(z_equals_Zd_temp) -> Logical Operator1/2
  Logical Operator2/1 -> z_goodenough/1

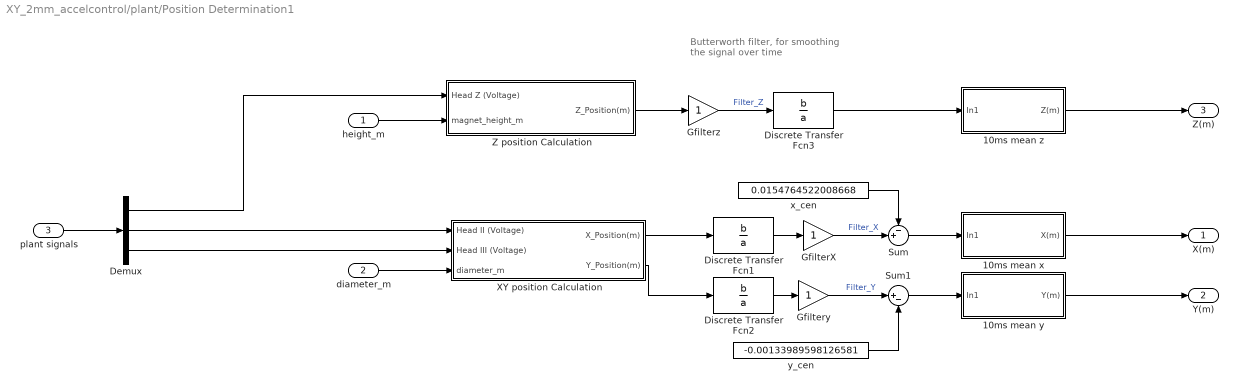
== system XY_2mm_accelcontrol/plant/Position Determination1 ==
  note: Butterworth filter, for smoothing the signal over time
  height_m : Inport
  diameter_m : Inport  Port=2
  plant signals : Inport  Port=3
  10ms mean x : Subsystem
  10ms mean y : Subsystem
  10ms mean z : Subsystem
  Demux : Demux  Outputs=3
  Discrete Transfer Fcn1 : DiscreteTransferFcn  Numerator=b  Denominator=a
  Discrete Transfer Fcn2 : DiscreteTransferFcn  Numerator=b  Denominator=a
  Discrete Transfer Fcn3 : DiscreteTransferFcn  Numerator=b  Denominator=a
  GfilterX : Gain
  Gfiltery : Gain
  Gfilterz : Gain
  Sum : Sum  Inputs=-+|
  Sum1 : Sum  Inputs=|+-
  XY position Calculation : Subsystem
  Z position Calculation : Subsystem
  x_cen : Constant  Value=0.0154764522008668
  y_cen : Constant  Value=-0.00133989598126581
  X(m) : Outport
  Y(m) : Outport  Port=2
  Z(m) : Outport  Port=3
  wires:
  Discrete Transfer Fcn2/1 -> Gfiltery/1
  Discrete Transfer Fcn1/1 -> GfilterX/1
  Gfilterz/1 -> Discrete Transfer Fcn3/1  "Filter_Z"
  GfilterX/1 -> Sum/2  "Filter_X"
  Gfiltery/1 -> Sum1/1  "Filter_Y"
  XY position Calculation/2(Y_Position(m)) -> Discrete Transfer Fcn2/1
  XY position Calculation/1(X_Position(m)) -> Discrete Transfer Fcn1/1
  Z position Calculation/1(Z_Position(m)) -> Gfilterz/1
  Discrete Transfer Fcn3/1 -> 10ms mean z/1(In1)
  x_cen/1 -> Sum/1
  y_cen/1 -> Sum1/2
  Sum/1 -> 10ms mean x/1(In1)
  Sum1/1 -> 10ms mean y/1(In1)
  height_m/1 -> Z position Calculation/2(magnet_height_m)
  diameter_m/1 -> XY position Calculation/3(diameter_m)
  plant signals/1 -> Demux/1
  Demux/1 -> Z position Calculation/1(Head Z (Voltage))
  Demux/2 -> XY position Calculation/1(Head II (Voltage))
  Demux/3 -> XY position Calculation/2(Head III (Voltage))
  10ms mean z/1(Z(m)) -> Z(m)/1
  10ms mean x/1(X(m)) -> X(m)/1
  10ms mean y/1(Y(m)) -> Y(m)/1

== system XY_2mm_accelcontrol/plant/output signal ==
  DS2004ADC_BL1 : rti2004lib/DS2004ADC_BL1  DSProperties=struct('RTI',struct('Version',uint32(1),'BlockType',struct('isSLSource',uint8(1),'isSLSink',uint8(1),'isHWSource',uint8(0),'isHWSink',uint8(1),'isSetup',uint8(0),'isInline',uint8(1),'isNonInline',uint8(0),'isInterrupt',uint8(0),'isChannelwise',uint8(1)),'IOBoardType','DS2004','UnitType','ADC','Identifier','ADC','DialogType','ML','BlockSet','NONE','SlaveProcessor','NONE'))  RTIBlockInterface=struct('InputPortsActive',0,'InputPortsWidth',int32(1),'InputPortsDataType',{{'SS_BOOLEAN'}},'InputPortsName',{{'Continue'}},'OutputPortsActive',[1 0],'OutputPortsWidth',int32([1 1]),'OutputPortsDataType',{{'SS_DOUBLE','SS_UINT8'}},'OutputPortsName',{{'ADC','Status'}},'DialogFcn','rti2004adcgui','SampleTime',{{-1}},'InitLevel',3,'IconTransparency','on','BlockDisplay',{{['DS2004 ADC\nBoard: 1\nChannel: 1'],'center'}},'BlockName',struct('Token',{{'DS2004ADC_BL1'}}))  RTIBlockParameters=struct('ADCSWStartDisable',{{0,'OFF',[0 1]}},'BoardNo',{{1,'OFF',[1 16]}},'ChannelNo',{{1,'OFF',[1 16]}},'ConversionMode',{{1,'OFF',[1 2]}},'SampleMode',{{1,'OFF',[1 2]}},'TriggerSource',{{1,'OFF',[1 5]}},'EdgePolarity',{{1,'OFF',[1 2]}},'ConversionTriggerSource',{{2,'OFF',[1 6]}},'ConversionEdgePolarity',{{1,'OFF',[1 2]}},'ConversionPeriod',{{1e-6,'OFF',[]}},'ConversionPeriodCheck',{{0,'OFF',[]}},'BurstTriggerSource',{{1,'OFF',[1 6]}},'BurstEdgePolarity',{{1,'OFF',[1 2]}},'BurstSize',{{10,'OFF',[]}},'BurstSizeCheck',{{0,'OFF',[]}},'DataSetOffset',{{0,'OFF',[]}},'DataSetOffsetCheck',{{0,'OFF',[]}},'DataSetLength',{{1,'OFF',[]}},'DataSetLengthCheck',{{0,'OFF',[]}},'ReadMode',{{1,'OFF',[1 2]}},'SampleTime',{{-1,'OFF',[-1 inf]}},'SampleTimeCheck',{{1,'OFF',[]}},'InputVoltageRange',{{2,'OFF',[1 2]}},'StatusPortEnable',{{0,'OFF',[0 1]}},'TLCFileName',{{'rti2004adc','OFF',[]}})  RTISFcnParameters=struct('ADCSWStartDisable','int32','BoardNo','int32','ChannelNo','int32','ConversionMode','int32','SampleMode','int32','TriggerSource','int32','EdgePolarity','int32','ConversionTriggerSource','int32','ConversionEdgePolarity','int32','ConversionPeriod','double','BurstTriggerSource','int32','BurstEdgePolarity','int32','BurstSize','int32','DataSetOffset','int32','DataSetLength','int32','ReadMode','int32','SampleTime','double','InputVoltageRange','int32','StatusPortEnable','int32','TLCFileName','char')  RTIBlockParaDefault=struct('ADCSWStartDisable',0,'BoardNo',1,'ChannelNo',1,'ConversionMode',1,'SampleMode',1,'TriggerSource',1,'EdgePolarity',1,'ConversionTriggerSource',2,'ConversionEdgePolarity',1,'ConversionPeriod',1e-6,'ConversionPeriodCheck',0,'BurstTriggerSource',1,'BurstEdgePolarity',1,'BurstSize',10,'BurstSizeCheck',0,'DataSetOffset',0,'DataSetOffsetCheck',0,'DataSetLength',1,'DataSetLengthCheck',0,'ReadMode',1,'SampleTime',-1,'SampleTimeCheck',1,'InputVoltageRange',2,'StatusPortEnable',0,'TLCFileName','rti2004adc')
  DS2004ADC_BL2 : rti2004lib/DS2004ADC_BL1  DSProperties=struct('RTI',struct('Version',uint32(1),'BlockType',struct('isSLSource',uint8(1),'isSLSink',uint8(1),'isHWSource',uint8(0),'isHWSink',uint8(1),'isSetup',uint8(0),'isInline',uint8(1),'isNonInline',uint8(0),'isInterrupt',uint8(0),'isChannelwise',uint8(1)),'IOBoardType','DS2004','UnitType','ADC','Identifier','ADC','DialogType','ML','BlockSet','NONE','SlaveProcessor','NONE'))  RTIBlockInterface=struct('InputPortsActive',0,'InputPortsWidth',int32(1),'InputPortsDataType',{{'SS_BOOLEAN'}},'InputPortsName',{{'Continue'}},'OutputPortsActive',[1 0],'OutputPortsWidth',int32([1 1]),'OutputPortsDataType',{{'SS_DOUBLE','SS_UINT8'}},'OutputPortsName',{{'ADC','Status'}},'DialogFcn','rti2004adcgui','SampleTime',{{-1}},'InitLevel',3,'IconTransparency','on','BlockDisplay',{{['DS2004 ADC\nBoard: 1\nChannel: 2'],'center'}},'BlockName',struct('Token',{{'DS2004ADC_BL1'}}))  RTIBlockParameters=struct('ADCSWStartDisable',{{0,'OFF',[0 1]}},'BoardNo',{{1,'OFF',[1 16]}},'ChannelNo',{{2,'OFF',[1 16]}},'ConversionMode',{{1,'OFF',[1 2]}},'SampleMode',{{1,'OFF',[1 2]}},'TriggerSource',{{1,'OFF',[1 5]}},'EdgePolarity',{{1,'OFF',[1 2]}},'ConversionTriggerSource',{{2,'OFF',[1 6]}},'ConversionEdgePolarity',{{1,'OFF',[1 2]}},'ConversionPeriod',{{'1e-006','OFF',[]}},'ConversionPeriodCheck',{{0,'OFF',[]}},'BurstTriggerSource',{{1,'OFF',[1 6]}},'BurstEdgePolarity',{{1,'OFF',[1 2]}},'BurstSize',{{'10','OFF',[]}},'BurstSizeCheck',{{0,'OFF',[]}},'DataSetOffset',{{'0','OFF',[]}},'DataSetOffsetCheck',{{0,'OFF',[]}},'DataSetLength',{{'1','OFF',[]}},'DataSetLengthCheck',{{0,'OFF',[]}},'ReadMode',{{1,'OFF',[1 2]}},'SampleTime',{{'-1','OFF',[-1 inf]}},'SampleTimeCheck',{{1,'OFF',[]}},'InputVoltageRange',{{2,'OFF',[1 2]}},'StatusPortEnable',{{0,'OFF',[0 1]}},'TLCFileName',{{'rti2004adc','OFF',[]}})  RTISFcnParameters=struct('ADCSWStartDisable','int32','BoardNo','int32','ChannelNo','int32','ConversionMode','int32','SampleMode','int32','TriggerSource','int32','EdgePolarity','int32','ConversionTriggerSource','int32','ConversionEdgePolarity','int32','ConversionPeriod','double','BurstTriggerSource','int32','BurstEdgePolarity','int32','BurstSize','int32','DataSetOffset','int32','DataSetLength','int32','ReadMode','int32','SampleTime','double','InputVoltageRange','int32','StatusPortEnable','int32','TLCFileName','char')  RTIBlockParaDefault=struct('ADCSWStartDisable',0,'BoardNo',1,'ChannelNo',1,'ConversionMode',1,'SampleMode',1,'TriggerSource',1,'EdgePolarity',1,'ConversionTriggerSource',2,'ConversionEdgePolarity',1,'ConversionPeriod',1e-6,'ConversionPeriodCheck',0,'BurstTriggerSource',1,'BurstEdgePolarity',1,'BurstSize',10,'BurstSizeCheck',0,'DataSetOffset',0,'DataSetOffsetCheck',0,'DataSetLength',1,'DataSetLengthCheck',0,'ReadMode',1,'SampleTime',-1,'SampleTimeCheck',1,'InputVoltageRange',2,'StatusPortEnable',0,'TLCFileName','rti2004adc')
  DS2004ADC_BL3 : rti2004lib/DS2004ADC_BL1  DSProperties=struct('RTI',struct('Version',uint32(1),'BlockType',struct('isSLSource',uint8(1),'isSLSink',uint8(1),'isHWSource',uint8(0),'isHWSink',uint8(1),'isSetup',uint8(0),'isInline',uint8(1),'isNonInline',uint8(0),'isInterrupt',uint8(0),'isChannelwise',uint8(1)),'IOBoardType','DS2004','UnitType','ADC','Identifier','ADC','DialogType','ML','BlockSet','NONE','SlaveProcessor','NONE'))  RTIBlockInterface=struct('InputPortsActive',0,'InputPortsWidth',int32(1),'InputPortsDataType',{{'SS_BOOLEAN'}},'InputPortsName',{{'Continue'}},'OutputPortsActive',[1 0],'OutputPortsWidth',int32([1 1]),'OutputPortsDataType',{{'SS_DOUBLE','SS_UINT8'}},'OutputPortsName',{{'ADC','Status'}},'DialogFcn','rti2004adcgui','SampleTime',{{-1}},'InitLevel',3,'IconTransparency','on','BlockDisplay',{{['DS2004 ADC\nBoard: 1\nChannel: 3'],'center'}},'BlockName',struct('Token',{{'DS2004ADC_BL1'}}))  RTIBlockParameters=struct('ADCSWStartDisable',{{0,'OFF',[0 1]}},'BoardNo',{{1,'OFF',[1 16]}},'ChannelNo',{{3,'OFF',[1 16]}},'ConversionMode',{{1,'OFF',[1 2]}},'SampleMode',{{1,'OFF',[1 2]}},'TriggerSource',{{1,'OFF',[1 5]}},'EdgePolarity',{{1,'OFF',[1 2]}},'ConversionTriggerSource',{{2,'OFF',[1 6]}},'ConversionEdgePolarity',{{1,'OFF',[1 2]}},'ConversionPeriod',{{'1e-006','OFF',[]}},'ConversionPeriodCheck',{{0,'OFF',[]}},'BurstTriggerSource',{{1,'OFF',[1 6]}},'BurstEdgePolarity',{{1,'OFF',[1 2]}},'BurstSize',{{'10','OFF',[]}},'BurstSizeCheck',{{0,'OFF',[]}},'DataSetOffset',{{'0','OFF',[]}},'DataSetOffsetCheck',{{0,'OFF',[]}},'DataSetLength',{{'1','OFF',[]}},'DataSetLengthCheck',{{0,'OFF',[]}},'ReadMode',{{1,'OFF',[1 2]}},'SampleTime',{{'-1','OFF',[-1 inf]}},'SampleTimeCheck',{{1,'OFF',[]}},'InputVoltageRange',{{2,'OFF',[1 2]}},'StatusPortEnable',{{0,'OFF',[0 1]}},'TLCFileName',{{'rti2004adc','OFF',[]}})  RTISFcnParameters=struct('ADCSWStartDisable','int32','BoardNo','int32','ChannelNo','int32','ConversionMode','int32','SampleMode','int32','TriggerSource','int32','EdgePolarity','int32','ConversionTriggerSource','int32','ConversionEdgePolarity','int32','ConversionPeriod','double','BurstTriggerSource','int32','BurstEdgePolarity','int32','BurstSize','int32','DataSetOffset','int32','DataSetLength','int32','ReadMode','int32','SampleTime','double','InputVoltageRange','int32','StatusPortEnable','int32','TLCFileName','char')  RTIBlockParaDefault=struct('ADCSWStartDisable',0,'BoardNo',1,'ChannelNo',1,'ConversionMode',1,'SampleMode',1,'TriggerSource',1,'EdgePolarity',1,'ConversionTriggerSource',2,'ConversionEdgePolarity',1,'ConversionPeriod',1e-6,'ConversionPeriodCheck',0,'BurstTriggerSource',1,'BurstEdgePolarity',1,'BurstSize',10,'BurstSizeCheck',0,'DataSetOffset',0,'DataSetOffsetCheck',0,'DataSetLength',1,'DataSetLengthCheck',0,'ReadMode',1,'SampleTime',-1,'SampleTimeCheck',1,'InputVoltageRange',2,'StatusPortEnable',0,'TLCFileName','rti2004adc')
  Head II (V) : Gain  Gain=10
  Head III (V) : Gain  Gain=10
  Head Z (V) : Gain  Gain=10
  Mux : Mux  Inputs=3
  plant signals : Outport
  wires:
  DS2004ADC_BL1/1 -> Head Z (V)/1
  DS2004ADC_BL2/1 -> Head III (V)/1
  DS2004ADC_BL3/1 -> Head II (V)/1
  Head Z (V)/1 -> Mux/1
  Head II (V)/1 -> Mux/2
  Head III (V)/1 -> Mux/3
  Mux/1 -> plant signals/1

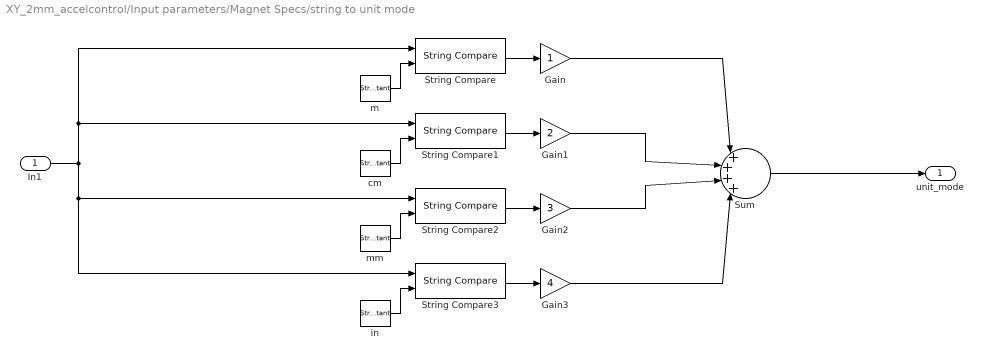
== system XY_2mm_accelcontrol/Input parameters/Magnet Specs/string to unit mode ==
  In1 : Inport
  Gain : Gain
  Gain1 : Gain  Gain=2
  Gain2 : Gain  Gain=3
  Gain3 : Gain  Gain=4
  String Compare{,1..3} (4 alike) : StringCompare
  Sum : Sum  Inputs=|++++|
  cm : StringConstant  String="\"cm\""
  in : StringConstant  String="\"in\""
  m : StringConstant  String="\"m\""
  mm : StringConstant  String="\"mm\""
  unit_mode : Outport
  wires:
  In1/1 -> String Compare3/1, String Compare2/1, String Compare/1, String Compare1/1
  m/1 -> String Compare/2
  cm/1 -> String Compare1/2
  mm/1 -> String Compare2/2
  in/1 -> String Compare3/2
  String Compare/1 -> Gain/1
  String Compare1/1 -> Gain1/1
  String Compare2/1 -> Gain2/1
  String Compare3/1 -> Gain3/1
  Sum/1 -> unit_mode/1
  Gain/1 -> Sum/1
  Gain1/1 -> Sum/2
  Gain2/1 -> Sum/3
  Gain3/1 -> Sum/4

== system XY_2mm_accelcontrol/RTI Data/RTI Data Store/RTI Data Store ==
  RTI Data Store : Subsystem  mask(RTI_DATA_STORE){}
      mask help:
      | RTI Data Store Block. This block is used by RTI to store internal model dependent data. Deleting this block will result in data loss.
      |
      | NEVER DELETE, COPY, OR MODIFY THIS BLOCK!
      mask Help:
      | RTI Data Store Block. This block is used by RTI to store internal model dependent data. Deleting this block will result in data loss.
      | 
      | NEVER DELETE, COPY, OR MODIFY THIS BLOCK!
      mask Display: text(0.5, 0.5, ' ', 'HorizontalAlignment', 'center');

== system XY_2mm_accelcontrol/get_plant_input/Z_1dctrl/Current2Vol1 ==
  note: Signal 1-2-4-6-5-1-2-3-4-3-5-6
  note: Amplifier takes an input voltage and outputs a current.
      | i = 0.355v , or v = 2.8169014i
      |
      | (where " i " is the desired current flowing through the coils, and " v " is the input voltage required to get this current!)
      |
      | (Notice that the v is multiplied by 0.1 before being sent to the dSPACE controller. Not sure why this is.)
  I : Inport
  Demux1 : Demux  Outputs=6
  Gain2 : Gain  Gain=.1
  Gain4 : Gain  Gain=2.8169014
  Mux2 : Mux  Inputs=6
  Mux3 : Mux  Inputs=6
  Mux5 : Mux  Inputs=2
  Saturation1 : Saturate  UpperLimit=8.2  LowerLimit=0
  Sum of Elements : Sum  Inputs=+
  V_discrepancies : Sum  Inputs=+-
  V_was_there_a_discrepancy? : simulink/Logic and Bit Operations/Compare To Zero  relop=~=  OutDataTypeStr=boolean
  I1toI6 : Outport
  I_exceeded : Outport  Port=2
  wires:
  Mux5/1 -> I1toI6/1
  I/1 -> Gain4/1
  Gain4/1 -> V_discrepancies/2, Saturation1/1
  Mux2/1 -> Mux5/1
  Saturation1/1 -> V_discrepancies/1, Gain2/1
  Gain2/1 -> Demux1/1  "4"
  Mux3/1 -> Mux5/2
  Demux1/1 -> Mux2/1, Mux2/6
  Demux1/2 -> Mux2/2, Mux3/1
  Demux1/4 -> Mux2/3, Mux3/3
  Demux1/6 -> Mux2/4, Mux3/6
  Demux1/5 -> Mux2/5, Mux3/5
  Demux1/3 -> Mux3/2, Mux3/4
  V_discrepancies/1 -> Sum of Elements/1
  Sum of Elements/1 -> V_was_there_a_discrepancy?/1
  V_was_there_a_discrepancy?/1 -> I_exceeded/1

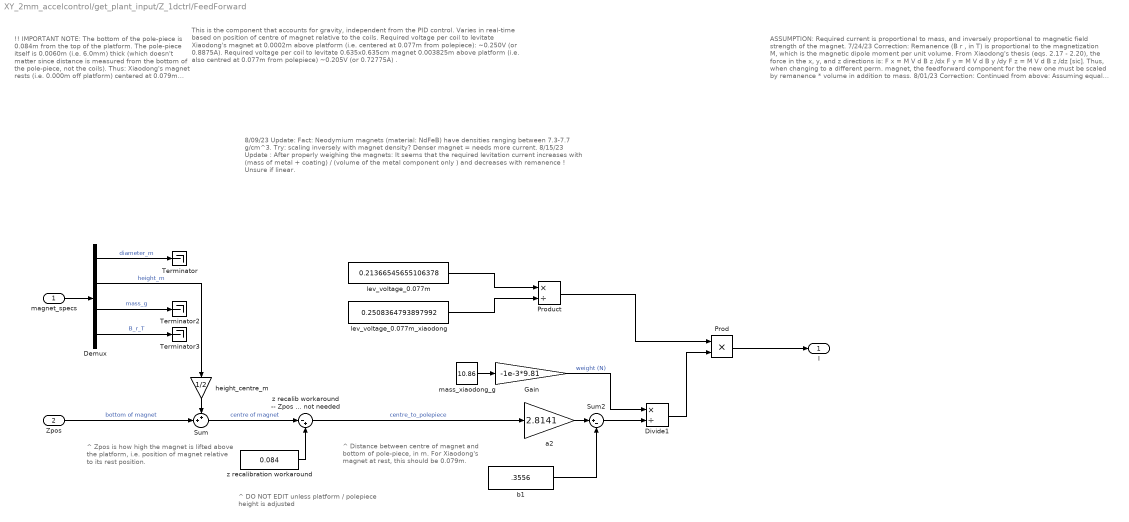
== system XY_2mm_accelcontrol/get_plant_input/Z_1dctrl/FeedForward ==
  note: ^ Zpos is how high the magnet is lifted above the platform, i.e. position of magnet relative to its rest position.
  note: 8/09/23 Update:
      |
      | Fact: Neodymium magnets (material: NdFeB) have densities ranging between 7.3-7.7 g/cm^3.
      | Try: scaling inversely with magnet density? Denser magnet = needs more current.
      |
      | 8/15/23 Update :
      | After properly weighing the magnets: It seems that the required levitation current increases with (mass of metal + coating) / (volume of the metal component only ) and decreases with remanence ! Unsure if linear.
  note: !! IMPORTANT NOTE:
      |
      | The bottom of the pole-piece is 0.084m from the top of the platform.
      | The pole-piece itself is 0.0060m (i.e. 6.0mm) thick (which doesn't matter since distance is measured from the bottom of the pole-piece, not the coils).
      |
      | Thus: Xiaodong's magnet rests (i.e. 0.000m off platform) centered at 0.079m from the polepiece (give or take 1mm due to deformity of the magnet).
  note: ASSUMPTION:
      | Required current is proportional to mass, and inversely proportional to magnetic field strength of the magnet.
      |
      | 7/24/23 Correction:
      | Remanence (B r , in T) is proportional to the magnetization M, which is the magnetic dipole moment per unit volume.
      |
      | From Xiaodong's thesis (eqs. 2.17 - 2.20), the force in the x, y, and z directions is:
      |
      | F x = M V d B z /dx
      |
      | F y = M V d B y /dy
      |
      | F z = M V d B z /dz [sic].
      |
      | Thus, when changing to a different perm. magnet, the feedforward component for the new one must be scaled by remanence * volume in addition to mass.
      |
      | 8/01/23 Correction:
      | Continued from above: Assuming equal density, volume scales with mass, and more volume = higher force produced but more mass = higher force required to levitate in the first place. Updated assumption: Any changes in mass will self-cancel due to corresponding changes in volume! (It's oversimplified and does not account for coating or the "b1" term to the left, but it's a step forward.)
  note: This is the component that accounts for gravity, independent from the PID control. Varies in real-time based on position of centre of magnet relative to the coils.
      |
      | Required voltage per coil to levitate Xiaodong's magnet at 0.0002m above platform (i.e. centered at 0.077m from polepiece): ~0.250V (or 0.8875A).
      |
      | Required voltage per coil to levitate 0.635x0.635cm magnet 0.003825m above platform (i.e. also centred at 0.077m from polepiece) ~0.205V (or 0.72775A) .
  note: ^ Distance between centre of magnet and bottom of pole-piece, in m.
      | For Xiaodong's magnet at rest, this should be 0.079m.
  note: ^ DO NOT EDIT unless platform / polepiece height is adjusted
  magnet_specs : Inport
  Zpos : Inport  Port=2
  Demux : Demux
  Divide1 : Product  Inputs=*/
  Gain : Gain  Gain=-1e-3*9.81
  Prod : Product  Inputs=**
  Product : Product  Inputs=*/
  Sum : Sum  Inputs=++|
  Sum2 : Sum  Inputs=|+-
  Terminator : Terminator
  Terminator2 : Terminator
  Terminator3 : Terminator
  a2 : Gain  Gain=2.8141
  b1 : Constant  Value=.3556
  height_centre_m : Gain  Gain=1/2
  lev_voltage_0.077m : Constant  Value=0.21366545655106378
  lev_voltage_0.077m_xiaodong : Constant  Value=0.2508364793897992
  mass_xiaodong_g : Constant  Value=10.86
  "z recalib workaround -- Zpos POSITIVE if not needed" : Sum  Inputs=|-+
  z recalibration workaround : Constant  Value=0.084
  I : Outport
  wires:
  a2/1 -> Sum2/1
  b1/1 -> Sum2/2
  Gain/1 -> Divide1/1  "weight (N)"
  Sum2/1 -> Divide1/2
  Divide1/1 -> Prod/2
  Prod/1 -> I/1
  "z recalib workaround -- Zpos POSITIVE if not needed"/1 -> a2/1  "centre_to_polepiece"
  z recalibration workaround/1 -> "z recalib workaround -- Zpos POSITIVE if not needed"/2
  Demux/1 -> Terminator/1  "diameter_m"
  magnet_specs/1 -> Demux/1
  Demux/3 -> Terminator2/1  "mass_g"
  Demux/4 -> Terminator3/1  "B_r_T"
  Zpos/1 -> Sum/2  "bottom of magnet"
  mass_xiaodong_g/1 -> Gain/1
  Demux/2 -> height_centre_m/1  "height_m"
  lev_voltage_0.077m/1 -> Product/1
  lev_voltage_0.077m_xiaodong/1 -> Product/2
  height_centre_m/1 -> Sum/1
  Sum/1 -> "z recalib workaround -- Zpos POSITIVE if not needed"/1  "centre of magnet"
  Product/1 -> Prod/1
